simulink model "Simulation_06"  (R2014a)
settings: Solver=ode45  StartTime=0.0  StopTime=10.0  RelTol=1e-3
settings Model: Creator=Dell  LastModifiedBy=Dell

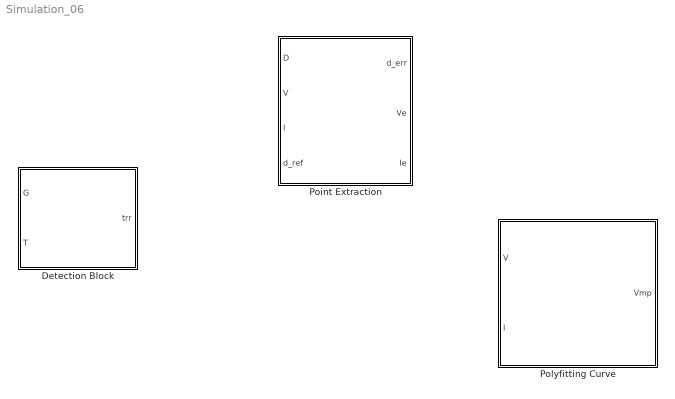
== system Simulation_06 ==
  Detection Block : MATLAB Function  TreatAsAtomicUnit=on
  Point Extraction : MATLAB Function  TreatAsAtomicUnit=on
  Polyfitting Curve : MATLAB Function  TreatAsAtomicUnit=on

== matlab function Simulation_06/Point Extraction ==
  data: D input; d_err output; V input; I input; d_ref input; Ve output; Ie output

function [d_err,Ve,Ie]= Curve_Fitting(D ,V , I, d_ref)
             
     

        persistent d_1 d_2 Vo Io io d_new
        dataType = 'double';
      
        if d_ref ~= d_new
                 vars = whos;
                vars = vars([vars.persistent]);
                varName = {vars.name};
                clear(varName{:});
                d_err=d_ref;
                Ve=[];
                Ie=[];
                return;
                
        end
    
        if isempty(Vo)
            Vo=0;
            Io=0;
            io=1;
            d_1=0;
            d_2=0;
            d_new=d_ref;
        end
        
        
        Vo
        Io
        d_ref 
        d_1
        d_2
      
                 if length(Vo)==3
                        Ve=Vo;
                        Ie=Io;
                        d_err=d_ref;
                        disp('Vector Array Limit Is Exceeded')

                        return;    
                 end

                 if length(Vo)<=2       
                        if D==d_1

                            disp('Adding Second Point in Array Vo and Io')
                            Vo(io)=V;
                            Io(io)=I;
                            d_2=d_ref - 0.2*d_ref;
                            d_err=d_2;     
                            io=io+1;

                        end

                        if D==d_ref
                            disp('Adding First Point in Array Vo and Io')
                            Vo(io)=V;
                            Io(io)=I;
                            d_1=d_ref + 0.2*d_ref;
                            d_err=d_1;
                            io=io+1;
                        end

                        if D==d_2
                            disp('Adding third Point in Array Vo and Io')
                            Vo(io)=V;
                            Io(io)=I;
                            d_err=d_2;
                            io=io+1;

                        end 
                 end
        
        Ve=Vo;
        Ie=Io;
end

== matlab function Simulation_06/Detection Block ==
  data: G input; trr output; T input
function trr= Detection(G,T)

     persistent G_ref
     dataType='double';
      
      if isempty(G)
         G_ref=1;
      end
      
      if G==G_ref
         
          y=0;
          G_ref=G;
          
      else
          
          y=1;
          G_ref=G;
          
      
      end 



end

== matlab function Simulation_06/Polyfitting Curve ==
  data: V input; Vmp output; I input
function Vmp = Polyfitting_Curve(V, I)
         
         Xo=V(1);
         X1=V(2);
         X2=V(3);
         
         Yo=I(1);
         Y1=I(2);
         Y2=I(3);
          
         a=0;
         b=0;
         c=0;
         d=0;
        
         t1=[Xo, X1, X2];
         t2=[Yo, Y1, Y2];
            
         
         X_t=polyfit(t1,t2,3);
         
         X_i=roots(X_t)
         
         Y_i=polyval(X_t,X_i(:))
         
         D_i=polyder(X_t)
         
         Y_new= roots(D_i)        
         
             
         Vmp=max(Y_i(:));
  
      
       
       
        
       
       

end
